simulink model "Modele_LQR_6DOF_EXPERIMENTATION"  (R2024b)
settings: Solver=VariableStepAuto  StartTime=0.0  StopTime=30  FixedStep=0.0001  RelTol=1e-3
values from neighbouring files (symbols this model uses):
  A_num = [0 0 0 0 0 0 0 0 0 0 0 0 ... (144 elements, 12x12)]    [Matrice_A_lineaire.mat]    (also in calcul_matrice_A_lineaire.m = double(A_num); resultats_stabilite.mat; testFinale.m = A_fcn(0, 0, 0, val_rll, val_ptc, val_yw, val_u, val_v, val_w; test_calcalV2.m = double(A_num))
  B = df_dcontrol    [Generate_PyMatrix.m]    (also in Parameters.m = -234.459; instabiliter_graphique.m = out.B_s.signals.values)
  Fx1 = -0.7071*force    (= -0.7071)    [Parameters.m]
  Fx2 = -0.7071*force    (= -0.7071)    [Parameters.m]
  Fx3 = 0    [Parameters.m]
  Fx4 = 0    [Parameters.m]
  Fx5 = 0    [Parameters.m]
  Fx6 = 0    [Parameters.m]
  Fx7 = 0.7071*force    (= 0.7071)    [Parameters.m]
  Fx8 = 0.7071*force    (= 0.7071)    [Parameters.m]
  Fy1 = 0.7071*force    (= 0.7071)    [Parameters.m]
  Fy2 = -0.7071*force    (= -0.7071)    [Parameters.m]
  Fy3 = 0    [Parameters.m]
  Fy4 = 0    [Parameters.m]
  Fy5 = 0    [Parameters.m]
  Fy6 = 0    [Parameters.m]
  Fy7 = 0.7071*force    (= 0.7071)    [Parameters.m]
  Fy8 = -0.7071*force    (= -0.7071)    [Parameters.m]
  Fz1 = 0    [Parameters.m]
  Fz2 = 0    [Parameters.m]
  Fz3 = -1*force    (= -1)    [Parameters.m]
  Fz4 = -1*force    (= -1)    [Parameters.m]
  Fz5 = -1*force    (= -1)    [Parameters.m]
  Fz6 = -1*force    (= -1)    [Parameters.m]
  Fz7 = 0    [Parameters.m]
  Fz8 = 0    [Parameters.m]
  I_x = 0.578    [Parameters.m]
  I_y = 0.645    [Parameters.m]
  I_z = 0.9366    [Parameters.m]
  lx1 = 0.2987    [Parameters.m]
  lx2 = 0.2987    [Parameters.m]
  lx3 = -0.1073    [Parameters.m]
  lx4 = -0.1073    [Parameters.m]
  lx5 = 0.1073    [Parameters.m]
  lx6 = 0.1073    [Parameters.m]
  lx7 = -0.2987    [Parameters.m]
  lx8 = -0.2987    [Parameters.m]
  ly1 = 0.2130    (= 0.213)    [Parameters.m]
  ly2 = -0.2130    (= -0.213)    [Parameters.m]
  ly3 = 0.2725    [Parameters.m]
  ly4 = -0.2725    [Parameters.m]
  ly5 = 0.2725    [Parameters.m]
  ly6 = -0.2725    [Parameters.m]
  ly7 = 0.2130    (= 0.213)    [Parameters.m]
  ly8 = -0.2130    (= -0.213)    [Parameters.m]
  lz1 = 0    [Parameters.m]
  lz2 = 0    [Parameters.m]
  lz3 = 0    [Parameters.m]
  lz4 = 0    [Parameters.m]
  lz5 = 0    [Parameters.m]
  lz6 = 0    [Parameters.m]
  lz7 = 0    [Parameters.m]
  lz8 = 0    [Parameters.m]
  m = 0.427    [Calcul_Inertie_Nouveau.m]    (also in Parameters.m = 23.9)
  Q_envoyer = Q_final(:,:,1)    [Parameters.m]
  W = mass*gravity    (= 234.459)    [Generate_PyMatrix.m]    (also in Parameters.m; calcul_damping.m)
  x_rb = 0    [Parameters.m]
  x_rg = 0    [Parameters.m]
  y_rb = 0    [Parameters.m]
  y_rg = 0    [Parameters.m]
  z_rb = 0    [Parameters.m]
  z_rg = 0    [Parameters.m]
undefined symbols (not defined in the file or in its folder): sigbuilder_block
libraries: simulink x12, sharedtransform x1, dspinverses x1, SignalEditorBlockLib x1
(part 3 of 3)

== matlab function Modele_LQR_6DOF_EXPERIMENTATION/Subsystem/MATLAB Function ==
  data: y input; angle output; x input; position input
function angle  = fcn(y, x, position)

persistent x_sub y_sub

% Initialiser la position actuelle si première exécution
if isempty(x_sub)
    x_sub = 0;
    y_sub = 0;
end
angle = 0;

if position(1) >= 1 && position(2) <= 1
    angle = pi/2;
end
if position(1) >= 1 && position(2) >= 1
    angle = pi;
end
if position(1) <= 1 && position(2) >= 1
    angle = pi/2;
end
if position(1) <= 1 && position(2) <= 1
    angle = 0;
end




% % Calculer le vecteur vers la commande
% dx = x - position(1);
% dy = y - position(2);
% 
% % Calculer l'angle avec atan2
% 
% angle = atan2(dy, dx);


% Normaliser entre 0 et 2*pi
% angle = mod(angle, 2*pi);




end

== matlab function Modele_LQR_6DOF_EXPERIMENTATION/Thrustherforces in newtons/MATLAB Function3 ==
  data: u input; y output
function y = Normalize(u)
y = (u-1500)*150/400;

== matlab function Modele_LQR_6DOF_EXPERIMENTATION/Thrustherforces in newtons/MATLAB Function4 ==
  data: u input; y output
function y = Normalize(u)
y = (u-1500)*150/400;

== matlab function Modele_LQR_6DOF_EXPERIMENTATION/Controller/MATLAB Function2 ==
  data: K input; u output; state input; target_state input
function u = State_error(K,state,target_state)
u = zeros(8,1);
u = -K*(state-target_state);
end

== matlab function Modele_LQR_6DOF_EXPERIMENTATION/Thrustherforces in newtons/MATLAB Function2 ==
  data: u input; tau output
function tau = fcn(u)
%#codegen
lookup =[...
    -40.0337   -1.0000
    -40.0337   -0.9750
    -40.0788   -0.9500
    -37.5428   -0.9250
    -36.6092   -0.9000
    -35.4971   -0.8750
    -33.7623   -0.8500
    -32.3835   -0.8250
    -31.2263   -0.8000
    -29.9809   -0.7750
    -28.5128   -0.7500
    -27.6234   -0.7250
    -26.5554   -0.7000
    -24.7765   -0.6750
    -23.1751   -0.6500
    -22.1522   -0.6250
    -21.3510   -0.6000
    -19.5280   -0.5750
    -18.4600   -0.5500
    -17.3480   -0.5250
    -16.1025   -0.5000
    -14.6345   -0.4750
    -13.0781   -0.4500
    -12.1877   -0.4250
    -10.9874   -0.4000
    -10.0528   -0.3750
    -8.8966   -0.3500
    -7.7404   -0.3250
    -6.8058   -0.3000
    -6.0497   -0.2750
    -5.1151   -0.2500
    -4.2698   -0.2250
    -3.4696   -0.2000
    -2.7135   -0.1750
    -1.8682   -0.1500
    -1.1121   -0.1250
    -0.5335   -0.1000
    -0.2667   -0.0750
    0   -0.0500
    0   -0.0250
    0         0
    0    0.0250
    0    0.0500
    0.5786    0.0750
    1.1121    0.1000
    1.8240    0.1250
    2.5801    0.1500
    3.4255    0.1750
    4.0923    0.2000
    5.1151    0.2250
    6.2272    0.2500
    7.0284    0.2750
    8.2739    0.3000
    9.2526    0.3250
    10.8089    0.3500
    12.2328    0.3750
    13.6558    0.4000
    14.9904    0.4250
    16.4585    0.4500
    17.7039    0.4750
    19.2161    0.5000
    20.5508    0.5250
    21.7521    0.5500
    23.6644    0.5750
    24.7324    0.6000
    26.4221    0.6250
    27.7126    0.6500
    29.6249    0.6750
    31.3156    0.7000
    32.8729    0.7250
    33.8065    0.7500
    34.2517    0.7750
    37.0534    0.8000
    38.6549    0.8250
    39.2776    0.8500
    41.1458    0.8750
    42.9257    0.9000
    44.7938    0.9250
    47.1062    0.9500
    48.0408    0.9750
    49.9531    1.0000];
%Thrustherforce in newtons.
tau = zeros(8,1);
tau(1) = interp1(lookup(:,2),lookup(:,1),u(1));
tau(2) = interp1(lookup(:,2),lookup(:,1),u(2));
tau(3) = interp1(lookup(:,2),lookup(:,1),u(3));
tau(4) = interp1(lookup(:,2),lookup(:,1),u(4));
tau(5) = interp1(lookup(:,2),lookup(:,1),u(5));
tau(6) = interp1(lookup(:,2),lookup(:,1),u(6));
tau(7) = interp1(lookup(:,2),lookup(:,1),u(7));
tau(8) = interp1(lookup(:,2),lookup(:,1),u(8));

end
